simulink model "SolarCellModelling"  (R2023a)
settings: Solver=VariableStepAuto  StartTime=0.0  StopTime=10.0  RelTol=1e-3
libraries: simulink x1
settings Model: Creator=paragmraw  LastModifiedBy=paragmraw

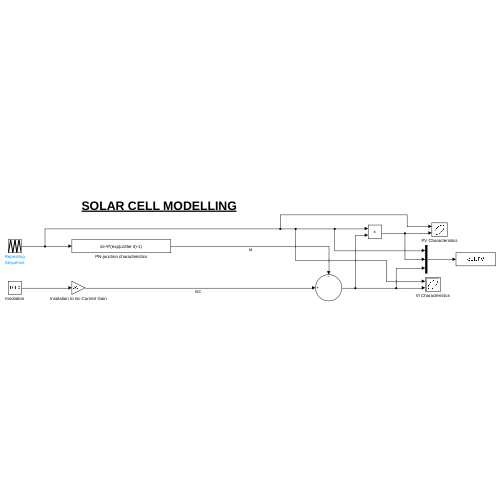
[thumbnail: Simulink's stored preview of the top-level diagram]
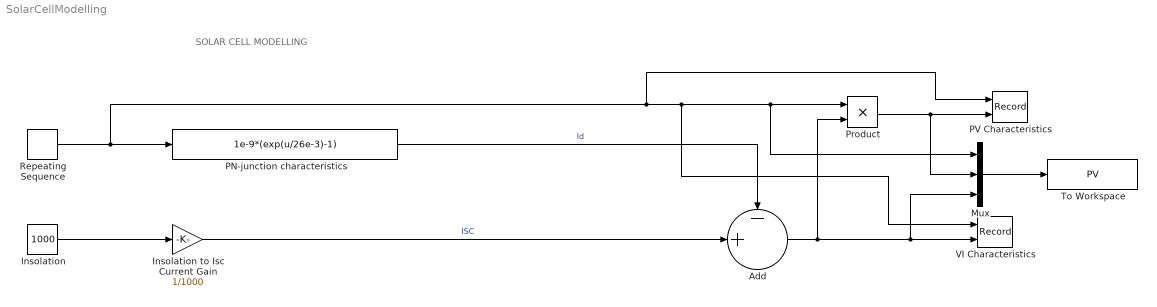
== system SolarCellModelling ==
  note: SOLAR CELL MODELLING
  Add : Sum  Inputs=-+|
  Insolation : Constant  Value=1000
  Insolation to Isc Current Gain : Gain  Gain=1/1000
  Mux : Mux  Inputs=3
  PN-junction characteristics : Fcn  Expr=1e-9*(exp(u/26e-3)-1)
  PV Characteristics : Record  FileSettingsInternal="{\"entries\":[{\"content\":{\"excelSettings\":{\"content\":{},\"type\":\"Streamout.ExcelSettings\"}},\"type\":\"Streamout.FileSettingStorage\",\"uuid\":\"\"}],\"packageUris\":[\"http:\\/\\/schema.mathworks.com\\/mf0\\/streamout_blocks\\/R2020a\"],\"version\":\"1.0\"}"  Layout=[1 1]  SignalsInternal="{\"entries\":[{\"content\":{\"signals\":[{\"content\":{\"blockPath\":[],\"dimensions\":[1],\"domain\":\"\",\"lineColor\":\"#a2142f\",\"plots\":[1],\"port\":1,\"signalID\":16,\"signalName\":\"XY Graph:1\"},\"type\":\"RecordBlkView.Signal\",\"uuid\":\"\"},{\"content\":{\"blockPath\":[],\"dimensions\":[1],\"domain\":\"\",\"lineColor\":\"#139fff\",\"plots\":[1],\"port\":2,\"signalID\":19,\"signalName\":\"XY Graph:2\"},\"type\":\"RecordBlkView.Signal\",\"uuid\":\"\"}]},\"type\":\"RecordBlkView.InputSignals\",\"uuid\":\"\"}],\"packageUris\":[\"http:\\/\\/schema.mathworks.com\\/mf0\\/streamout_blocks\\/R2020a\"],\"version\":\"1.0\"}"  VisualizationBindings="{\"xyplotplugin\":{\"info\":[{\"series\":[{\"bindingParametersList\":[{\"parameter\":\"X-Axis\",\"signalID\":16,\"signalName\":\"XY Graph:1\"},{\"parameter\":\"Y-Axis\",\"signalID\":19,\"signalName\":\"XY Graph:2\"}],\"seriesID\":1596}],\"subplotID\":1}]}}"  CompatibilityTag=XY
  Product : Product
  Repeating Sequence : simulink/Sources/Repeating Sequence  rep_seq_t=[0 1 2]  rep_seq_y=[-0.1 0.6 -0.1]
  To Workspace : ToWorkspace  VariableName=PV  SaveFormat=Structure With Time  SampleTime=-1
  VI Characteristics : Record  FileSettingsInternal="{\"entries\":[{\"content\":{\"excelSettings\":{\"content\":{},\"type\":\"Streamout.ExcelSettings\"}},\"type\":\"Streamout.FileSettingStorage\",\"uuid\":\"\"}],\"packageUris\":[\"http:\\/\\/schema.mathworks.com\\/mf0\\/streamout_blocks\\/R2020a\"],\"version\":\"1.0\"}"  Layout=[1 1]  SignalsInternal="{\"entries\":[{\"content\":{\"signals\":[{\"content\":{\"blockPath\":[],\"dimensions\":[1],\"domain\":\"\",\"lineColor\":\"#a2142f\",\"plots\":[1],\"port\":1,\"signalID\":24,\"signalName\":\"XY Graph:1\"},\"type\":\"RecordBlkView.Signal\",\"uuid\":\"\"},{\"content\":{\"blockPath\":[],\"dimensions\":[1],\"domain\":\"\",\"lineColor\":\"#139fff\",\"plots\":[1],\"port\":2,\"signalID\":27,\"signalName\":\"XY Graph:2\"},\"type\":\"RecordBlkView.Signal\",\"uuid\":\"\"}]},\"type\":\"RecordBlkView.InputSignals\",\"uuid\":\"\"}],\"packageUris\":[\"http:\\/\\/schema.mathworks.com\\/mf0\\/streamout_blocks\\/R2020a\"],\"version\":\"1.0\"}"  VisualizationBindings="{\"xyplotplugin\":{\"info\":[{\"series\":[{\"bindingParametersList\":[{\"parameter\":\"X-Axis\",\"signalID\":24,\"signalName\":\"XY Graph:1\"},{\"parameter\":\"Y-Axis\",\"signalID\":27,\"signalName\":\"XY Graph:2\"}],\"seriesID\":64596}],\"subplotID\":1}]}}"  CompatibilityTag=XY
  wires:
  Repeating Sequence/1 -> PV Characteristics/1, VI Characteristics/1, Mux/1, Product/1, PN-junction characteristics/1
  Insolation/1 -> Insolation to Isc Current Gain/1
  PN-junction characteristics/1 -> Add/1  "Id"
  Insolation to Isc Current Gain/1 -> Add/2  "ISC"
  Add/1 -> Mux/3, VI Characteristics/2, Product/2
  Product/1 -> PV Characteristics/2, Mux/2
  Mux/1 -> To Workspace/1
